simulink model "Modell_V6"  (R2017a)
settings: Solver=ode45  StartTime=0.0  StopTime=2  RelTol=1e-3
values from neighbouring files (symbols this model uses):
  mK = [0.891414391377 1.27328256447 -8.10548044357 -0.387729574757 0.892333044237 1.27380762349 -8.10779333021 -0.3875762591 0.893168625263 1.27430179537 -8.10985852649 -0.387416063485 ... (3112 elements, 4x778)]    [Ergebnisse.mat]    (also in berechneK.m = reshape(mK,n,size(mK,2)/n))
  stPendel =     [Ergebnisse.mat]    (also in V6.m = ladePendel())
  stTraj =     [Ergebnisse.mat]    (also in RiccatiDGL.m = RiccatiCache.stTraj; V6.m = berechneTrajektorie(stPendel, traj.Q, traj.R,Tend))
  vTK = [0 0.0003003003003 0.000600600600601 0.000900900900901 0.0012012012012 0.0015015015015 0.0018018018018 0.0021021021021 0.0024024024024 0.0027027027027 0.003003003003 0.0033033033033 ... (778 elements, 778x1)]    [Ergebnisse.mat]    (also in berechneK.m = flipud(vTK))
  x0 = [0 0 0 0]    [Ergebnisse.mat]    (also in V6.m = [0;0;0;0])
settings Model: Creator=asacakli  LastModifiedBy=Ali Kerem Sacakli
settings DataIOCC: LimitDataPoints=on  SaveFormat=Array
settings OptimizationCC: BlockReduction=off  BooleanDataType=off  LifeSpan=inf
settings DebuggingCC: SaveWithParameterizedLinksMsg=none  UnderspecifiedInitializationDetection=Classic  MergeDetectMultiDrivingBlocksExec=none  SignalResolutionControl=TryResolveAllWithWarning  SFUnexpectedBacktrackingDiag=warning  SFNoUnconditionalDefaultTransitionDiag=warning  SFExecutionAtInitializationDiag=none
settings HardwareCC: ProdBitPerPointer=32  ProdBitPerSizeT=32  ProdBitPerPtrDiffT=32  ProdLargestAtomicFloat=None  ProdIntDivRoundTo=Undefined  ProdEndianess=Unspecified  ProdWordSize=32  ProdHWDeviceType=32-bit Generic  TargetUnknown=on
settings ModelReferenceCC: PropagateSignalLabelsOutOfModel=off
settings GRTTargetCC: TargetLangStandard=C89/C90 (ANSI)  GeneratePreprocessorConditionals=Disable all
settings ConfigComp: CovMetricSettings=dw  CovHtmlReporting=on  CovSaveCumulativeToWorkspaceVar=on  CovSaveSingleToWorkspaceVar=on  CovExternalEMLEnable=off  CovSFcnEnable=off

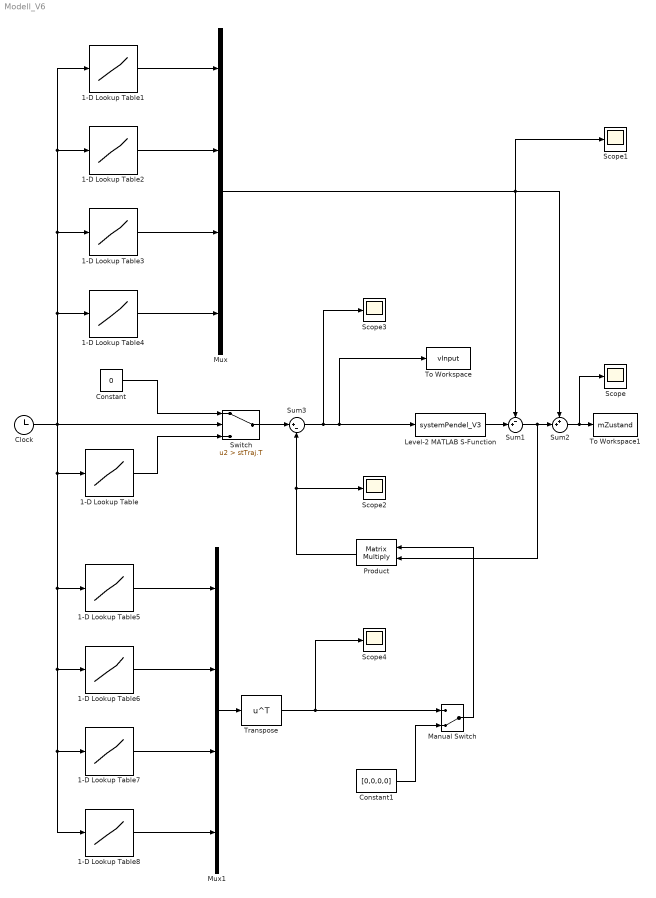
== system Modell_V6 ==
  1-D Lookup Table : Lookup_n-D  NumberOfTableDimensions=1  BreakpointsForDimension1=stTraj.vT  Table=stTraj.vU  InterpMethod=Cubic spline  ExtrapMethod=Clip  InternalRulePriority=Speed  RndMeth=Simplest  InputSameDT=on
  1-D Lookup Table1 : Lookup_n-D  NumberOfTableDimensions=1  BreakpointsForDimension1=stTraj.vT  Table=stTraj.mX(1,:)  InterpMethod=Cubic spline  ExtrapMethod=Clip  InternalRulePriority=Speed  RndMeth=Simplest  InputSameDT=on
  1-D Lookup Table2 : Lookup_n-D  NumberOfTableDimensions=1  BreakpointsForDimension1=stTraj.vT  Table=stTraj.mX(2,:)  InterpMethod=Cubic spline  ExtrapMethod=Clip  InternalRulePriority=Speed  RndMeth=Simplest  InputSameDT=on
  1-D Lookup Table3 : Lookup_n-D  NumberOfTableDimensions=1  BreakpointsForDimension1=stTraj.vT  Table=stTraj.mX(3,:)  InterpMethod=Cubic spline  ExtrapMethod=Clip  InternalRulePriority=Speed  RndMeth=Simplest  InputSameDT=on
  1-D Lookup Table4 : Lookup_n-D  NumberOfTableDimensions=1  BreakpointsForDimension1=stTraj.vT  Table=stTraj.mX(4,:)  InterpMethod=Cubic spline  ExtrapMethod=Clip  InternalRulePriority=Speed  RndMeth=Simplest  InputSameDT=on
  1-D Lookup Table5 : Lookup_n-D  NumberOfTableDimensions=1  BreakpointsForDimension1=vTK  Table=mK(1,:)  InterpMethod=Cubic spline  ExtrapMethod=Clip  InternalRulePriority=Speed  RndMeth=Simplest  InputSameDT=on
  1-D Lookup Table6 : Lookup_n-D  NumberOfTableDimensions=1  BreakpointsForDimension1=vTK  Table=mK(2,:)  InterpMethod=Cubic spline  ExtrapMethod=Clip  InternalRulePriority=Speed  RndMeth=Simplest  InputSameDT=on
  1-D Lookup Table7 : Lookup_n-D  NumberOfTableDimensions=1  BreakpointsForDimension1=vTK  Table=mK(3,:)  InterpMethod=Cubic spline  ExtrapMethod=Clip  InternalRulePriority=Speed  RndMeth=Simplest  InputSameDT=on
  1-D Lookup Table8 : Lookup_n-D  NumberOfTableDimensions=1  BreakpointsForDimension1=vTK  Table=mK(4,:)  InterpMethod=Cubic spline  ExtrapMethod=Clip  InternalRulePriority=Speed  RndMeth=Simplest  InputSameDT=on
  Clock : Clock
  Constant : Constant  Value=0
  Constant1 : Constant  Value=[0,0,0,0]  VectorParams1D=off
  Level-2 MATLAB S-Function : M-S-Function  FunctionName=systemPendel_V3  Parameters=stPendel,x0
  Manual Switch : ManualSwitch  CurrentSetting=0
  Mux : Mux
  Mux1 : Mux
  Product : Product  Inputs=**  Multiplication=Matrix(*)
  Scope{,1..4} (5 alike) : Scope
  Sum1 : Sum  Inputs=-+|
  Sum2 : Sum  Inputs=++|
  Sum3 : Sum  Inputs=|+-
  Switch : Switch  Criteria=u2 > Threshold  Threshold=stTraj.T
  To Workspace : ToWorkspace  VariableName=vInput  SaveFormat=Timeseries  SampleTime=-1
  To Workspace1 : ToWorkspace  VariableName=mZustand  SaveFormat=Timeseries  SampleTime=-1
  Transpose : Math  Operator=transpose  SaturateOnIntegerOverflow=on
  wires:
  Sum2/1 -> Scope/1, To Workspace1/1
  1-D Lookup Table/1 -> Switch/3
  Constant/1 -> Switch/1
  1-D Lookup Table1/1 -> Mux/1
  1-D Lookup Table2/1 -> Mux/2
  1-D Lookup Table3/1 -> Mux/3
  1-D Lookup Table4/1 -> Mux/4
  Clock/1 -> 1-D Lookup Table2/1, 1-D Lookup Table1/1, 1-D Lookup Table3/1, 1-D Lookup Table4/1, 1-D Lookup Table5/1, 1-D Lookup Table8/1, 1-D Lookup Table7/1, 1-D Lookup Table6/1, 1-D Lookup Table/1, Switch/2
  1-D Lookup Table5/1 -> Mux1/1
  1-D Lookup Table6/1 -> Mux1/2
  1-D Lookup Table7/1 -> Mux1/3
  1-D Lookup Table8/1 -> Mux1/4
  Switch/1 -> Sum3/1
  Sum3/1 -> Scope3/1, To Workspace/1, Level-2 MATLAB S-Function/1
  Product/1 -> Scope2/1, Sum3/2
  Level-2 MATLAB S-Function/1 -> Sum1/2
  Mux/1 -> Scope1/1, Sum1/1, Sum2/1
  Constant1/1 -> Manual Switch/2
  Mux1/1 -> Transpose/1
  Transpose/1 -> Manual Switch/1, Scope4/1
  Sum1/1 -> Product/2, Sum2/2
  Manual Switch/1 -> Product/1
